simulink model "IBC_open"  (R2019b)
settings: Solver=VariableStepAuto  StartTime=0.0  StopTime=0.02  RelTol=1e-3
InitFcn:
  | Load=2;
  | C=370e-6;
  | L1=1000e-6;
  | L2=1000e-6*(1+normrnd(0,0.05,[1,1]));
  | L3=1000e-6*(1+normrnd(0,0.05,[1,1]));
  | alp=1-0.5;
  | V=12;
libraries: powerlib x23, simulink x12, dspsigops x4
settings Model: SimulationMode=accelerator  Creator=29721  LastModifiedBy=29721

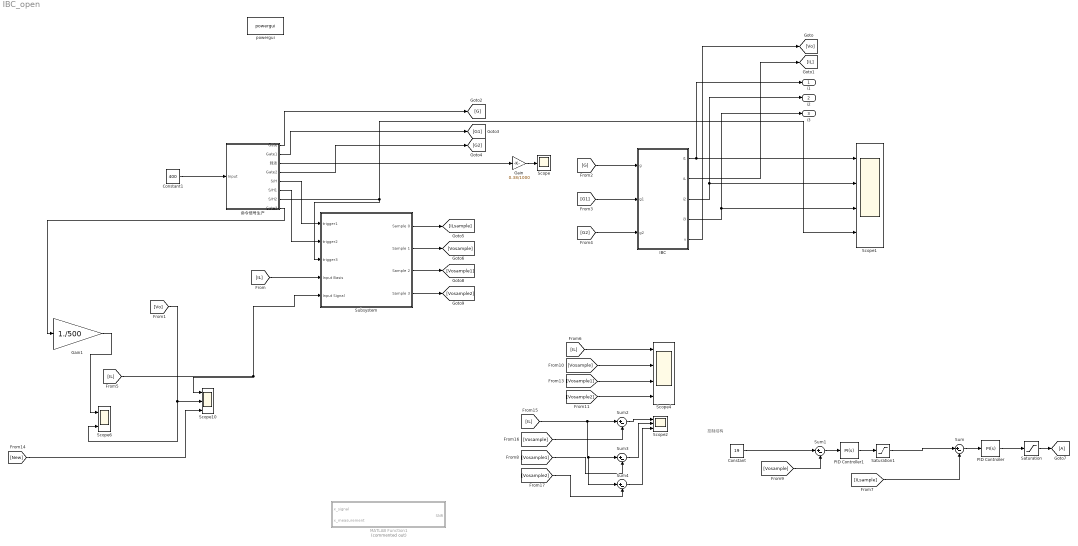
== system IBC_open ==
  note: 控制结构
  Constant : Constant  Value=19
  Constant1 : Constant  Value=400
  Gain : Gain  Gain=0.38/1000
  Gain1 : Gain  Gain=1./500
  IBC : Subsystem  mask{Vin=V, C=C, Load=Load, L1=L1, L2=L1, L3=L1}
  MATLAB Function1 : MATLAB Function  Commented=on  TreatAsAtomicUnit=on
  PID Controller : simulink/Continuous/PID Controller  Controller=PI  Form=Parallel  TimeDomain=Continuous-time  SampleTime=-1  IntegratorMethod=Forward Euler  FilterMethod=Forward Euler  ControllerParametersSource=internal  P=140  I=186020.6134968  D=0  UseFilter=on  N=100  TunerSelectOption=Transfer Function Based (PID Tuner App)  InitialConditionSource=internal  InitialConditionForIntegrator=0  InitialConditionForFilter=0  DifferentiatorICPrevScaledInput=0  ExternalReset=none  TrackingMode=off  Kt=1  LimitOutput=off  UpperSaturationLimit=inf  LowerSaturationLimit=-inf  LinearizeAsGain=on  AntiWindupMode=none  Kb=1  POutMin=[]  POutMax=[]  IOutMin=[]  IOutMax=[]  DOutMin=[]  DOutMax=[]  NOutMin=[]  NOutMax=[]  SumOutMin=[]  SumOutMax=[]  SaturationOutMin=[]  SaturationOutMax=[]  PParamMin=[]  PParamMax=[]  IParamMin=[]  IParamMax=[]  DParamMin=[]  DParamMax=[]  NParamMin=[]  NParamMax=[]  KbParamMin=[]  KbParamMax=[]  KtParamMin=[]  KtParamMax=[]  KbOutMin=[]  KbOutMax=[]  KtOutMin=[]  KtOutMax=[]  IntegratorOutMin=[]  IntegratorOutMax=[]  FilterOutMin=[]  FilterOutMax=[]  SumI1OutMin=[]  SumI1OutMax=[]  SumI2OutMin=[]  SumI2OutMax=[]  SumI3OutMin=[]  SumI3OutMax=[]  SumI4OutMin=[]  SumI4OutMax=[]  SumDOutMin=[]  SumDOutMax=[]  DifferentiatorOutMin=[]  DifferentiatorOutMax=[]  FilterDiffOutCoefMin=[]  FilterDiffOutCoefMax=[]  ReciprocalOutMin=[]  ReciprocalOutMax=[]  SumDenOutMin=[]  SumDenOutMax=[]  SumNumOutMin=[]  SumNumOutMax=[]  DivideOutMin=[]  DivideOutMax=[]  IntegratorContinuousStateAttributes=''  IntegratorStateMustResolveToSignalObject=off  IntegratorRTWStateStorageClass=Auto  FilterContinuousStateAttributes=''  FilterStateMustResolveToSignalObject=off  FilterRTWStateStorageClass=Auto  ParallelPVariant=InternalParameters  IdealPVariant=Disabled  IVariant=InternalParameters  DVariant=Disabled  IntegratorVariant=Continuous  SatVariant=Disabled  AWVariant=Passthrough  PCopyVariant=Disabled  TRVariant=Disabled  FdbkBlocksVariant=Forward  IdealPFdbkVariant=Disabled  SatFdbkVariant=Disabled  DerivativeFilterVariant=Disabled  NVariant=Disabled  NCopyVariant=Disabled_SignalSpec  FilterICVariant=Disabled  IntegratorICVariant=InternalICs  ExternalResetVariant=Disabled  TRSumVariant=Passthrough  SumFdbkVariant=Disabled  SumVariant=Sum_PI
  PID Controller1 : simulink/Continuous/PID Controller  Controller=PI  Form=Parallel  TimeDomain=Continuous-time  SampleTime=-1  IntegratorMethod=Forward Euler  FilterMethod=Forward Euler  ControllerParametersSource=internal  P=0.01  I=500  D=0  UseFilter=on  N=100  TunerSelectOption=Transfer Function Based (PID Tuner App)  InitialConditionSource=internal  InitialConditionForIntegrator=0  InitialConditionForFilter=0  DifferentiatorICPrevScaledInput=0  ExternalReset=none  TrackingMode=off  Kt=1  LimitOutput=off  UpperSaturationLimit=inf  LowerSaturationLimit=-inf  LinearizeAsGain=on  AntiWindupMode=none  Kb=1  POutMin=[]  POutMax=[]  IOutMin=[]  IOutMax=[]  DOutMin=[]  DOutMax=[]  NOutMin=[]  NOutMax=[]  SumOutMin=[]  SumOutMax=[]  SaturationOutMin=[]  SaturationOutMax=[]  PParamMin=[]  PParamMax=[]  IParamMin=[]  IParamMax=[]  DParamMin=[]  DParamMax=[]  NParamMin=[]  NParamMax=[]  KbParamMin=[]  KbParamMax=[]  KtParamMin=[]  KtParamMax=[]  KbOutMin=[]  KbOutMax=[]  KtOutMin=[]  KtOutMax=[]  IntegratorOutMin=[]  IntegratorOutMax=[]  FilterOutMin=[]  FilterOutMax=[]  SumI1OutMin=[]  SumI1OutMax=[]  SumI2OutMin=[]  SumI2OutMax=[]  SumI3OutMin=[]  SumI3OutMax=[]  SumI4OutMin=[]  SumI4OutMax=[]  SumDOutMin=[]  SumDOutMax=[]  DifferentiatorOutMin=[]  DifferentiatorOutMax=[]  FilterDiffOutCoefMin=[]  FilterDiffOutCoefMax=[]  ReciprocalOutMin=[]  ReciprocalOutMax=[]  SumDenOutMin=[]  SumDenOutMax=[]  SumNumOutMin=[]  SumNumOutMax=[]  DivideOutMin=[]  DivideOutMax=[]  IntegratorContinuousStateAttributes=''  IntegratorStateMustResolveToSignalObject=off  IntegratorRTWStateStorageClass=Auto  FilterContinuousStateAttributes=''  FilterStateMustResolveToSignalObject=off  FilterRTWStateStorageClass=Auto  ParallelPVariant=InternalParameters  IdealPVariant=Disabled  IVariant=InternalParameters  DVariant=Disabled  IntegratorVariant=Continuous  SatVariant=Disabled  AWVariant=Passthrough  PCopyVariant=Disabled  TRVariant=Disabled  FdbkBlocksVariant=Forward  IdealPFdbkVariant=Disabled  SatFdbkVariant=Disabled  DerivativeFilterVariant=Disabled  NVariant=Disabled  NCopyVariant=Disabled_SignalSpec  FilterICVariant=Disabled  IntegratorICVariant=InternalICs  ExternalResetVariant=Disabled  TRSumVariant=Passthrough  SumFdbkVariant=Disabled  SumVariant=Sum_PI
  Saturation : Saturate  UpperLimit=900  LowerLimit=100
  Saturation1 : Saturate  UpperLimit=5  LowerLimit=0
  Scope : Scope
  Scope1 : Scope  NumInputPorts=4
  Scope10 : Scope  NumInputPorts=3
  Scope2 : Scope  NumInputPorts=3
  Scope4 : Scope  NumInputPorts=4
  Scope6 : Scope  NumInputPorts=2
  Subsystem : Subsystem
  Sum{,1..4} (5 alike) : Sum  Inputs=|+-
  powergui : powerlib/powergui  Priority=1  SimulationMode=Discrete  SampleTime=2.5e-8  frequency=60  Iterations=50  frequencyindice=0  Pbase=100e6  ErrMax=1e-4  UnitsV=kV  UnitsW=MW  buscounter=0  FunctionMessages=off  echomessages=off  EnableUseOfTLC=off  CurrentSourceSwitches=off  DisableSnubberDevices=off  DisableRonSwitches=off  DisableVfSwitches=off  DisplayEquations=off  AutomaticDiscreteSolvers=off  SolverType=Tustin/Backward Euler (TBE)  Interpol=off  ExternalGateDelay=off  methode=off  Ts=100  x0status=blocks  SPID=on  SwTol=0  HookPort=off  NonlinearTolerance=1e-4  nMaxIteration=100  ContinueOnMaxIteration=off  RestoreLinks=warning  ResistiveCurrentMeasurement=off  Frange=[0:2:500]  Ylog=off  Xlog=on  ShowGrid=off  save=off  variable=ZData  structure=0  ZoomFFT=off  StartTime=0.0  cycles=1  DisplayStyle=1  fundamental=60  FreqAxis=off  MaxFrequency=1000  frequencyindicesteady=1  RmsSteady=1  display=off
      settings: SourceProductName=Simscape Electrical
  命令信号生产 : Subsystem  mask{Fs=10e3}
      mask prompts: Fs "swicthing frequency"
  i1 : Outport
  i2 : Outport  Port=2
  i3 : Outport  Port=3
  wires:
  Sum1/1 -> PID Controller1/1
  [Vosample1] -> Scope4/3
  [ILsample] -> Sum/2
  [New] -> Scope10/3
  [Vosample2] -> Scope4/4
  [IL] -> Subsystem/5(Input Signal), Scope10/1
  Constant/1 -> Sum1/1
  Sum/1 -> PID Controller/1
  PID Controller/1 -> Saturation/1
  Saturation1/1 -> Sum/1
  [Vo] -> Scope6/2, Scope10/2
  [Vosample] -> Scope4/2
  Gain1/1 -> Scope6/1
  命令信号生产/7(S/H2) -> Subsystem/3(trigger3), Scope1/4
  Saturation/1 -> [A]
  [Vosample] -> Sum1/2
  命令信号生产/8(Gate3) -> Gain1/1
  PID Controller1/1 -> Saturation1/1
  [G] -> IBC/1(g)
  [G1] -> IBC/2(g1)
  [G2] -> IBC/3(g2)
  IBC/1(i1) -> i1/1, Scope1/1
  IBC/2(iL) -> [IL]
  IBC/3(i2) -> Scope1/2, i2/1
  IBC/4(i3) -> Scope1/3, i3/1
  IBC/5(v) -> [Vo]
  Constant1/1 -> 命令信号生产/1(Input)
  命令信号生产/1(Gate) -> [G]
  命令信号生产/2(Gate1) -> [G1]
  命令信号生产/4(Gate2) -> [G2]
  命令信号生产/3(载波) -> Gain/1
  Gain/1 -> Scope/1
  [Vosample] -> Sum2/2
  [IL] -> Sum4/1, Sum3/1, Sum2/1
  Sum2/1 -> Scope2/1
  [Vosample1] -> Sum3/2
  Sum3/1 -> Scope2/2
  [Vosample2] -> Sum4/2
  Sum4/1 -> Scope2/3
  命令信号生产/5(S/H) -> Subsystem/1(trigger1)
  命令信号生产/6(S/H1) -> Subsystem/2(trigger2)
  [IL] -> Subsystem/4(Input Basis)
  Subsystem/1(Sample 0) -> [ILsample]
  Subsystem/2(Sample 1) -> [Vosample]
  Subsystem/3(Sample 2) -> [Vosample1]
  Subsystem/4(Sample 3) -> [Vosample2]
  [IL] -> Scope4/1

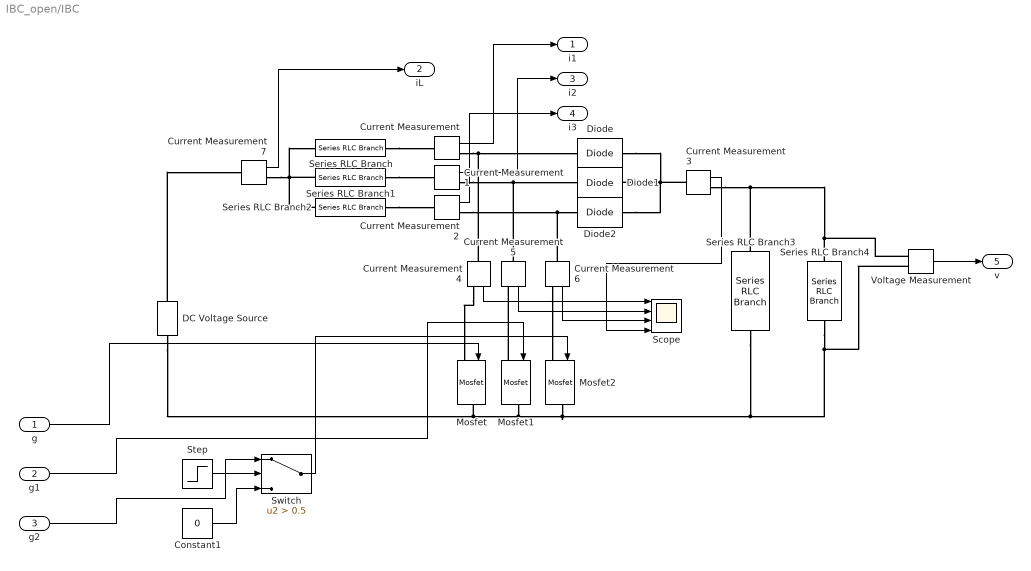
== system IBC_open/IBC ==
  g : Inport
  g1 : Inport  Port=2
  g2 : Inport  Port=3
  Constant1 : Constant  Value=0
  Current Measurement{,1..7} (8 alike) : powerlib/Measurements/Current Measurement  PhasorSimulation=off  OutputType=Complex  PSBequivalent=0
      settings: SourceProductName=Simscape Electrical
  DC Voltage Source : powerlib/Electrical Sources/DC Voltage Source  Amplitude=V  Measurements=None
      settings: SourceProductName=Simscape Electrical
  Diode : powerlib/Power Electronics/Diode  Ron=0.001  Lon=0  Vf=0.8  IC=0  UseSnubber=0  Rs=inf  Cs=250e-9  Measurements=off
      settings: SourceProductName=Simscape Electrical
  Diode1 : powerlib/Power Electronics/Diode  Ron=0.001  Lon=0  Vf=0.8  IC=0  UseSnubber=0  Rs=inf  Cs=250e-9  Measurements=off
      settings: SourceProductName=Simscape Electrical
  Diode2 : powerlib/Power Electronics/Diode  Ron=0.001  Lon=0  Vf=0.8  IC=0  UseSnubber=0  Rs=inf  Cs=250e-9  Measurements=off
      settings: SourceProductName=Simscape Electrical
  Mosfet : powerlib/Power Electronics/Mosfet  Ron=0.1  Lon=0  Rd=0.01  Vfd=0  IC=0  Rs=1e5  Cs=inf  Measurements=off
      settings: SourceProductName=Simscape Electrical
  Mosfet1 : powerlib/Power Electronics/Mosfet  Ron=0.1  Lon=0  Rd=0.01  Vfd=0  IC=0  Rs=1e5  Cs=inf  Measurements=off
      settings: SourceProductName=Simscape Electrical
  Mosfet2 : powerlib/Power Electronics/Mosfet  Ron=0.1  Lon=0  Rd=0.01  Vfd=0  IC=0  Rs=1e5  Cs=inf  Measurements=off
      settings: SourceProductName=Simscape Electrical
  Scope : Scope  NumInputPorts=4
  Series RLC Branch : powerlib/Elements/Series RLC Branch  LConnTagsString=__new0  RConnTagsString=__new0  BranchType=L  Resistance=1  Inductance=L1  SetiL0=off  InitialCurrent=0  Capacitance=1e-6  Setx0=off  InitialVoltage=0  Measurements=None
      settings: SourceProductName=Simscape Electrical
  Series RLC Branch1 : powerlib/Elements/Series RLC Branch  LConnTagsString=__new0  RConnTagsString=__new0  BranchType=L  Resistance=1  Inductance=L2  SetiL0=off  InitialCurrent=0  Capacitance=1e-6  Setx0=off  InitialVoltage=0  Measurements=None
      settings: SourceProductName=Simscape Electrical
  Series RLC Branch2 : powerlib/Elements/Series RLC Branch  LConnTagsString=__new0  RConnTagsString=__new0  BranchType=L  Resistance=1  Inductance=L3  SetiL0=off  InitialCurrent=0  Capacitance=1e-6  Setx0=off  InitialVoltage=0  Measurements=None
      settings: SourceProductName=Simscape Electrical
  Series RLC Branch3 : powerlib/Elements/Series RLC Branch  LConnTagsString=__new0  RConnTagsString=__new0  BranchType=RC  Resistance=0.1  Inductance=1e-3  SetiL0=off  InitialCurrent=0  Capacitance=C  Setx0=off  InitialVoltage=0  Measurements=None
      settings: SourceProductName=Simscape Electrical
  Series RLC Branch4 : powerlib/Elements/Series RLC Branch  LConnTagsString=__new0  RConnTagsString=__new0  BranchType=R  Resistance=Load  Inductance=1e-3  SetiL0=off  InitialCurrent=0  Capacitance=C  Setx0=off  InitialVoltage=0  Measurements=None
      settings: SourceProductName=Simscape Electrical
  Step : Step  Time=0.01  Before=1  After=0  SampleTime=0
  Switch : Switch  Criteria=u2 > Threshold  Threshold=0.5
  Voltage Measurement : powerlib/Measurements/Voltage Measurement  PhasorSimulation=off  OutputType=Complex  PSBequivalent=0
      settings: SourceProductName=Simscape Electrical
  i1 : Outport
  iL : Outport  Port=2
  i2 : Outport  Port=3
  i3 : Outport  Port=4
  v : Outport  Port=5
  wires:
  Voltage Measurement/1 -> v/1
  g2/1 -> Switch/1
  Current Measurement/1 -> i1/1
  g/1 -> Mosfet/1
  Current Measurement2/1 -> i3/1
  Step/1 -> Switch/2
  Current Measurement3/1 -> Scope/4
  g1/1 -> Mosfet1/1
  Switch/1 -> Mosfet2/1
  Current Measurement1/1 -> i2/1
  Constant1/1 -> Switch/3
  Current Measurement7/1 -> iL/1
  Current Measurement6/1 -> Scope/3
  Current Measurement4/1 -> Scope/1
  Current Measurement5/1 -> Scope/2
  connections:
  DC Voltage Source/LConn1 -- Mosfet1/RConn1 -- Mosfet2/RConn1 -- Series RLC Branch4/RConn1 -- Voltage Measurement/LConn2 -- Series RLC Branch3/RConn1 -- Mosfet/RConn1
  Current Measurement1/RConn1 -- Diode1/LConn1 -- Current Measurement5/LConn1
  Current Measurement3/LConn1 -- Diode2/RConn1 -- Diode/RConn1 -- Diode1/RConn1
  Current Measurement7/RConn1 -- Series RLC Branch2/LConn1 -- Series RLC Branch1/LConn1 -- Series RLC Branch/LConn1
  Current Measurement4/RConn1 -- Mosfet/LConn1
  Current Measurement3/RConn1 -- Series RLC Branch3/LConn1 -- Series RLC Branch4/LConn1 -- Voltage Measurement/LConn1
  Current Measurement/RConn1 -- Diode/LConn1 -- Current Measurement4/LConn1
  Current Measurement2/RConn1 -- Current Measurement6/LConn1 -- Diode2/LConn1
  Series RLC Branch1/RConn1 -- Current Measurement1/LConn1
  Series RLC Branch/RConn1 -- Current Measurement/LConn1
  DC Voltage Source/RConn1 -- Current Measurement7/LConn1
  Series RLC Branch2/RConn1 -- Current Measurement2/LConn1
  Mosfet1/LConn1 -- Current Measurement5/RConn1
  Current Measurement6/RConn1 -- Mosfet2/LConn1

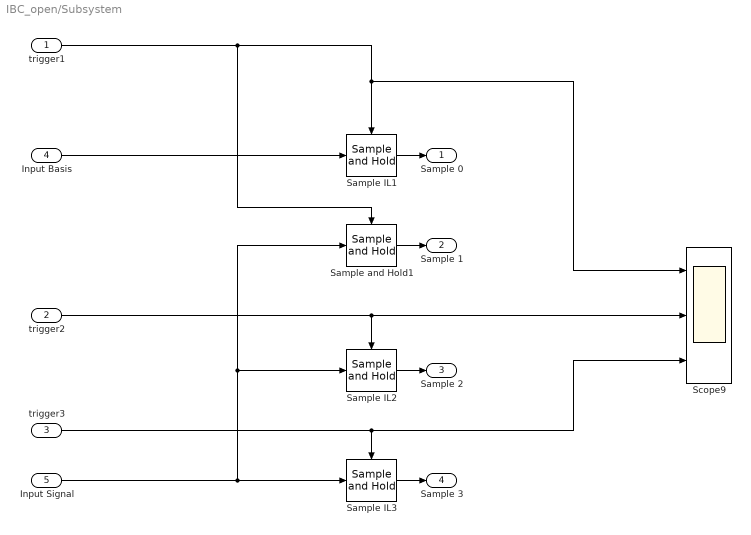
== system IBC_open/Subsystem ==
  trigger1 : Inport
  trigger2 : Inport  Port=2
  trigger3 : Inport  Port=3
  Input Basis : Inport  Port=4
  Input Signal : Inport  Port=5
  Sample IL1 : dspsigops/Sample and Hold  trig=Rising edge  initCond=0  latchinput=off
  Sample IL2 : dspsigops/Sample and Hold  trig=Rising edge  initCond=0  latchinput=off
  Sample IL3 : dspsigops/Sample and Hold  trig=Rising edge  initCond=0  latchinput=off
  Sample and Hold1 : dspsigops/Sample and Hold  trig=Rising edge  initCond=0  latchinput=off
  Scope9 : Scope  NumInputPorts=3
  Sample 0 : Outport
  Sample 1 : Outport  Port=2
  Sample 2 : Outport  Port=3
  Sample 3 : Outport  Port=4
  wires:
  trigger3/1 -> Sample IL3/Trigger, Scope9/3
  Input Signal/1 -> Sample and Hold1/1, Sample IL2/1, Sample IL3/1
  Sample IL3/1 -> Sample 3/1
  trigger1/1 -> Scope9/1, Sample IL1/Trigger, Sample and Hold1/Trigger
  trigger2/1 -> Sample IL2/Trigger, Scope9/2
  Sample IL2/1 -> Sample 2/1
  Input Basis/1 -> Sample IL1/1
  Sample IL1/1 -> Sample 0/1
  Sample and Hold1/1 -> Sample 1/1

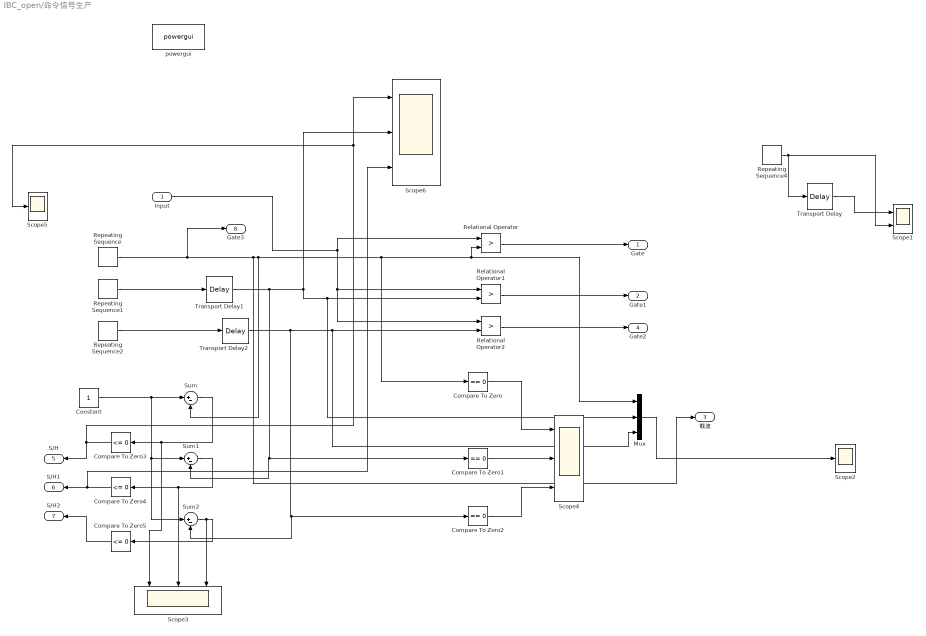
== system IBC_open/命令信号生产 ==
  Input : Inport
  Compare To Zero : simulink/Logic and Bit Operations/Compare To Zero  relop===  OutDataTypeStr=boolean
  Compare To Zero1 : simulink/Logic and Bit Operations/Compare To Zero  relop===  OutDataTypeStr=boolean
  Compare To Zero2 : simulink/Logic and Bit Operations/Compare To Zero  relop===  OutDataTypeStr=boolean
  Compare To Zero3 : simulink/Logic and Bit Operations/Compare To Zero  relop=<=  OutDataTypeStr=boolean
  Compare To Zero4 : simulink/Logic and Bit Operations/Compare To Zero  relop=<=  OutDataTypeStr=boolean
  Compare To Zero5 : simulink/Logic and Bit Operations/Compare To Zero  relop=<=  OutDataTypeStr=boolean
  Constant : Constant
  Mux : Mux  Inputs=3
  Relational Operator : RelationalOperator  Operator=>  OutDataTypeStr=boolean  RndMeth=Simplest
  Relational Operator1 : RelationalOperator  Operator=>  OutDataTypeStr=boolean  RndMeth=Simplest
  Relational Operator2 : RelationalOperator  Operator=>  OutDataTypeStr=boolean  RndMeth=Simplest
  Repeating Sequence : simulink/Sources/Repeating Sequence  rep_seq_t=[0 1./Fs./2 1./Fs]  rep_seq_y=[0 1000 0]
  Repeating Sequence1 : simulink/Sources/Repeating Sequence  rep_seq_t=[1./Fs./3 5./Fs./6 4./Fs./3]  rep_seq_y=[0 1000 0]
  Repeating Sequence2 : simulink/Sources/Repeating Sequence  rep_seq_t=[2./Fs./3 7./Fs./6 5./Fs./3]  rep_seq_y=[0 1000 0]
  Repeating Sequence4 : simulink/Sources/Repeating Sequence  rep_seq_t=[0 1./100e3./2 1./100e3]  rep_seq_y=[0 1000 0]
  Scope1 : Scope  NumInputPorts=2
  Scope2 : Scope
  Scope3 : Scope  NumInputPorts=3
  Scope4 : Scope  NumInputPorts=3
  Scope5 : Scope
  Scope6 : Scope  NumInputPorts=3
  Sum : Sum  Inputs=|+-
  Sum1 : Sum  Inputs=|+-
  Sum2 : Sum  Inputs=|+-
  Transport Delay : TransportDelay  DelayTime=1./100e3./3
  Transport Delay1 : TransportDelay  DelayTime=1./Fs./3
  Transport Delay2 : TransportDelay  DelayTime=2./Fs./3
  powergui : powerlib/powergui  Priority=1  SimulationMode=Discrete  SampleTime=2.5e-8  frequency=60  Iterations=50  frequencyindice=60  Pbase=100e6  ErrMax=1e-4  UnitsV=kV  UnitsW=MW  buscounter=0  FunctionMessages=off  echomessages=off  EnableUseOfTLC=off  CurrentSourceSwitches=off  DisableSnubberDevices=off  DisableRonSwitches=off  DisableVfSwitches=off  DisplayEquations=off  AutomaticDiscreteSolvers=off  SolverType=Tustin/Backward Euler (TBE)  Interpol=off  ExternalGateDelay=off  methode=off  Ts=100  x0status=blocks  SPID=on  SwTol=0  HookPort=off  NonlinearTolerance=1e-4  nMaxIteration=100  ContinueOnMaxIteration=off  RestoreLinks=warning  ResistiveCurrentMeasurement=off  Frange=[0:2:500]  Ylog=off  Xlog=on  ShowGrid=off  save=off  variable=ZData  structure=0  ZoomFFT=off  StartTime=0.0  cycles=1  DisplayStyle=1  fundamental=60  FreqAxis=off  MaxFrequency=1000  frequencyindicesteady=1  RmsSteady=1  display=off
      settings: SourceProductName=Simscape Electrical
  Gate : Outport
  Gate1 : Outport  Port=2
  载波 : Outport  Port=3
  Gate2 : Outport  Port=4
  S/H : Outport  Port=5
  S/H1 : Outport  Port=6
  S/H2 : Outport  Port=7
  Gate3 : Outport  Port=8
  wires:
  Input/1 -> Relational Operator1/1, Relational Operator2/1, Relational Operator/1
  Compare To Zero/1 -> Scope4/1
  Relational Operator/1 -> Gate/1
  Repeating Sequence1/1 -> Transport Delay1/1
  Relational Operator1/1 -> Gate1/1
  Repeating Sequence2/1 -> Transport Delay2/1
  Repeating Sequence/1 -> Gate3/1, Mux/1, Relational Operator/2, Compare To Zero/1, Sum/2, 载波/1
  Relational Operator2/1 -> Gate2/1
  Repeating Sequence4/1 -> Transport Delay/1, Scope1/2
  Transport Delay/1 -> Scope1/1
  Mux/1 -> Scope2/1
  Transport Delay1/1 -> Sum1/2, Compare To Zero1/1, Scope6/2, Mux/2, Relational Operator1/2
  Compare To Zero1/1 -> Scope4/2
  Compare To Zero2/1 -> Scope4/3
  Sum/1 -> Scope3/1, Compare To Zero3/1
  Sum1/1 -> Compare To Zero4/1, Scope3/2
  Transport Delay2/1 -> Sum2/2, Compare To Zero2/1, Mux/3, Relational Operator2/2
  Sum2/1 -> Scope3/3, Compare To Zero5/1
  Constant/1 -> Sum2/1, Sum1/1, Sum/1
  Compare To Zero3/1 -> Scope6/1, Scope5/1, S/H/1
  Compare To Zero4/1 -> Scope6/3, S/H1/1
  Compare To Zero5/1 -> S/H2/1

== matlab function IBC_open/MATLAB Function1 ==
  data: x_signal input; SNR output; x_measurement input
function SNR = SNR_calculte(x_signal,x_measurement)
%================== Calculate the SNR ===================%
x_noise = x_measurement-x_signal;
% Calculate the power of the signal and noise
Ps = sum(x_signal.^2)./length(x_signal);
Pn = sum(x_noise.^2)./length(x_noise);
% Calculate the SNR
SNR = 10*log10(Ps/Pn);
